simulink model "simpleprocess"  (Simulink 7.4)
settings: Solver=ode45  StartTime=0.0  StopTime=15  RelTol=1e-3
settings Model: Creator=Alex  LastModifiedBy=Alex

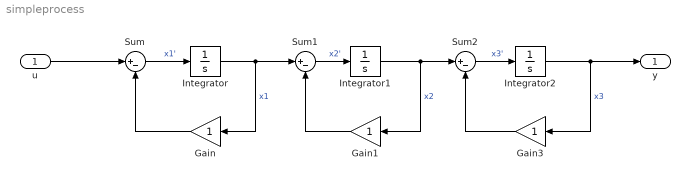
== system simpleprocess ==
  u : Inport  OutDataType=fixdt(1, 16)  OutScaling=2^0
  Gain : Gain  ParameterDataType=fixdt(1, 16)  ParameterScaling=2^0  OutDataType=fixdt(1, 16)  OutScaling=2^0
  Gain1 : Gain  ParameterDataType=fixdt(1, 16)  ParameterScaling=2^0  OutDataType=fixdt(1, 16)  OutScaling=2^0
  Gain3 : Gain  ParameterDataType=fixdt(1, 16)  ParameterScaling=2^0  OutDataType=fixdt(1, 16)  OutScaling=2^0
  Integrator : Integrator
  Integrator1 : Integrator
  Integrator2 : Integrator
  Sum : Sum  Inputs=|+-  OutDataType=fixdt(1, 16)  OutScaling=2^0
  Sum1 : Sum  Inputs=|+-  OutDataType=fixdt(1, 16)  OutScaling=2^0
  Sum2 : Sum  Inputs=|+-  OutDataType=fixdt(1, 16)  OutScaling=2^0
  y : Outport  OutDataType=fixdt(1, 16)  OutScaling=2^0
  wires:
  Gain/1 -> Sum/2
  Sum/1 -> Integrator/1  "x1'"
  Integrator2/1 -> Gain3/1, y/1  "x3"
  Integrator/1 -> Sum1/1, Gain/1  "x1"
  Sum1/1 -> Integrator1/1  "x2'"
  Integrator1/1 -> Sum2/1, Gain1/1  "x2"
  Sum2/1 -> Integrator2/1  "x3'"
  Gain1/1 -> Sum1/2
  Gain3/1 -> Sum2/2
  u/1 -> Sum/1
